simulink model "rtd_prova"  (R2019a)
settings: Solver=VariableStepAuto  StartTime=0.0  StopTime=10.0  RelTol=1e-3
undefined symbols (not defined in the file): sigbuilder_block
settings Model: Creator=francoseminara  LastModifiedBy=andreabiondo
settings DataIOCC: ReturnWorkspaceOutputs=off
settings DebuggingCC: ArithmeticOperatorsInVariantConditions=warning

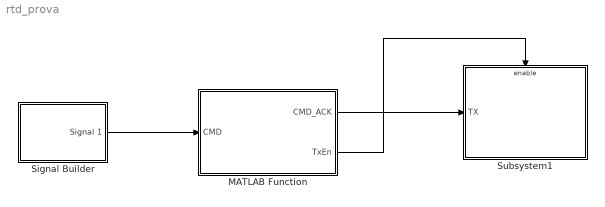
== system rtd_prova ==
  MATLAB Function : MATLAB Function  TreatAsAtomicUnit=on
  Signal Builder : Subsystem  Tag=STV Subsys  LoadFcn=sigbuilder_block('load');  StartFcn=sigbuilder_block('start');  StopFcn=sigbuilder_block('stop');  ClipboardFcn=sigbuilder_block('clipboard');  mask(Sigbuilder block){tuvar=[0:10]}
      mask help: Simulink:masks:SigbuilderBlock_MD
      mask init:
      | if ~strcmp(get_param(bdroot(gcbh),'SimulationStatus'),'stopped') tuvar = sigbuilder_block('maskInit'); end
      settings: CopyFcn=sigbuilder_block('copy');  DeleteFcn=sigbuilder_block('delete');  ModelCloseFcn=sigbuilder_block('modelClose');  PreSaveFcn=sigbuilder_block('preSave');  PauseFcn=sigbuilder_block('pause');  ContinueFcn=sigbuilder_block('continue');  NameChangeFcn=sigbuilder_block('namechange');  OpenFcn=sigbuilder_block('open',[437.6 199.2 550.4 400 ]);  CloseFcn=sigbuilder_block('close');
      mask Display: plot(0, 0, 100, 100,[2, 2, 32, 32, 2], [68, 8, 8, 68, 68],[32, 2], [38, 38], [32, 19, 2],[53, 60, 44], [32, 17, 17, 2],[16, 16, 31, 31]);txt = getActiveGroup(gcbh);text(2, 100, txt,'verticalAlignment', 'top');
  Subsystem1 : Subsystem
  wires:
  Signal Builder/1(Signal 1) -> MATLAB Function/1(CMD)
  MATLAB Function/2(TxEn) -> Subsystem1/Enable
  MATLAB Function/1(CMD_ACK) -> Subsystem1/1(TX)

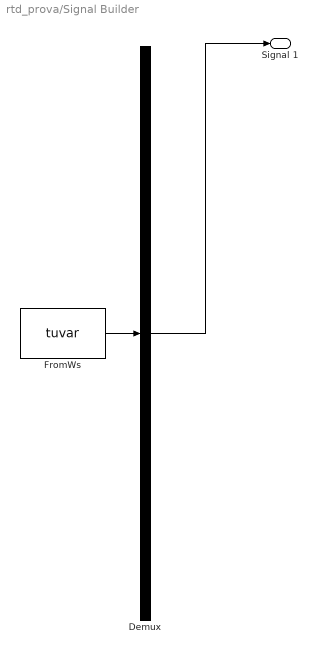
== system rtd_prova/Signal Builder ==
  Demux : Demux  Tag=STV Demux  Outputs=1
  FromWs : FromWorkspace  Tag=STV FromWs  VariableName=tuvar  SampleTime=0
      SigBuilderData=|
      | common.afterFinalStr = 'Extrapolate'
      | common.sampleTime = 0
      | dataSet.timeRange = [0 10]
      | dataSet.name = 'Group 1'
      | sbobj.Groups.Name = 'Group 1'
      | sbobj.Groups.Signals.Name = 'Signal 1'
      | sbobj.Groups.Signals.XData = [0 2 2 4 4 5 5 6 6 10]
      | sbobj.Groups.Signals.YData = [0 0 1 1 0 0 2 2 0 0]
  Signal 1 : Outport  Tag=STV Outport
  wires:
  Demux/1 -> Signal 1/1
  FromWs/1 -> Demux/1

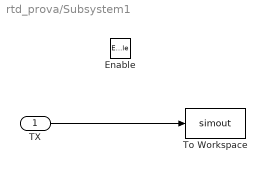
== system rtd_prova/Subsystem1 ==
  TX : Inport
  Enable : EnablePort
  To Workspace : ToWorkspace  VariableName=simout  SaveFormat=Timeseries  SampleTime=-1
  wires:
  TX/1 -> To Workspace/1

== matlab function rtd_prova/MATLAB Function ==
  data: CMD input; CMD_ACK output; TxEn output
function [CMD_ACK, TxEn] = fcn(CMD)


persistent check
if isempty(check)
    check = 0;
end

CMD_ACK = 0;
TxEn = 0;

%First push, send acknowledge 
if CMD == 1 && check==0
    CMD_ACK = 1;
    TxEn = 1;
    check = 1;
end

%Second push, send acknowledge, RTD ON
if CMD == 2 && check == 1
    CMD_ACK = 2;
    TxEn = 1;
    check = 2;
end
